simulink model "Model_plant"  (R2022a)
settings: Solver=VariableStepAuto  StartTime=0.0  StopTime=10  RelTol=1e-3
values from neighbouring files (symbols this model uses):
  init = [theta_m_init; theta_l_init; thetadot_m_init; thetadot_l_init; Ia_init]    [ELEN90064_Project_Parameters.m]
undefined symbols (not defined in the file or in its folder): denC, denG, numC, numG
settings Model: Creator=Admin  LastModifiedBy=yang

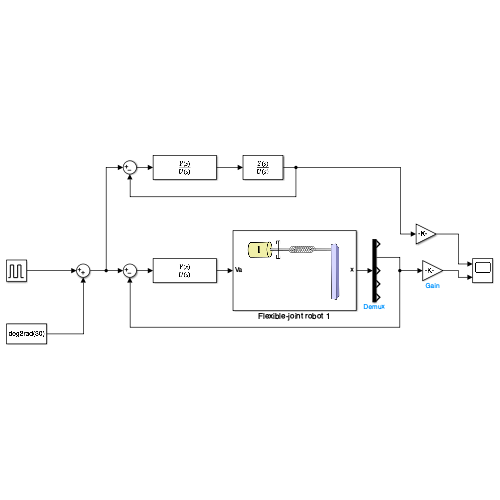
[thumbnail: Simulink's stored preview of the top-level diagram]
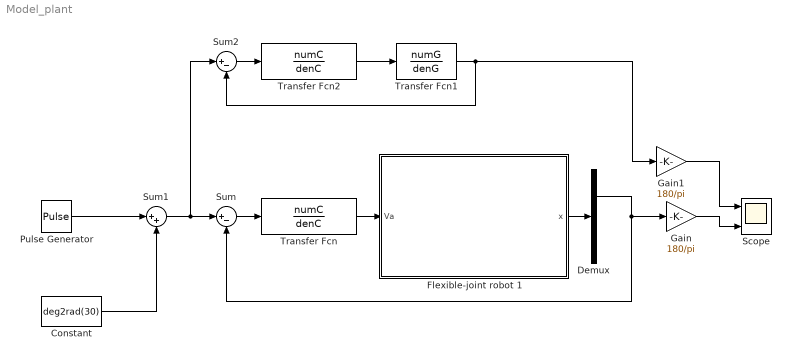
== system Model_plant ==
  Constant : Constant  Value=deg2rad(30)
  Demux : Demux  Outputs=5
  Flexible-joint robot 1 : Subsystem
      mask Display: image('$imagefile'); % Use "Edit Image" on toolstrip to change.
  Gain : Gain  Gain=180/pi
  Gain1 : Gain  Gain=180/pi
  Pulse Generator : DiscretePulseGenerator  PulseType=Time based  Amplitude=deg2rad(30)  Period=5  PulseWidth=50
  Scope : Scope  NumInputPorts=2
  Sum : Sum  Inputs=|+-
  Sum1 : Sum  Inputs=|++
  Sum2 : Sum  Inputs=|+-
  Transfer Fcn : TransferFcn  Numerator=numC  Denominator=denC
  Transfer Fcn1 : TransferFcn  Numerator=numG  Denominator=denG
  Transfer Fcn2 : TransferFcn  Numerator=numC  Denominator=denC
  wires:
  Sum/1 -> Transfer Fcn/1
  Pulse Generator/1 -> Sum1/1
  Constant/1 -> Sum1/2
  Gain/1 -> Scope/2
  Transfer Fcn/1 -> Flexible-joint robot 1/1(Va)
  Flexible-joint robot 1/1(x) -> Demux/1
  Demux/2 -> Gain/1, Sum/2
  Transfer Fcn1/1 -> Gain1/1, Sum2/2
  Sum1/1 -> Sum2/1, Sum/1
  Sum2/1 -> Transfer Fcn2/1
  Transfer Fcn2/1 -> Transfer Fcn1/1
  Gain1/1 -> Scope/1

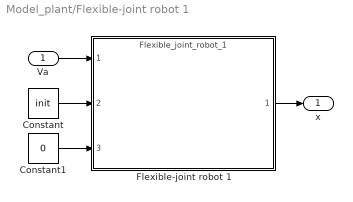
== system Model_plant/Flexible-joint robot 1 ==
  Va : Inport
  Constant : Constant  Value=init
  Constant1 : Constant  Value=0
  Flexible-joint robot 1 : ModelReference  ModelNameDialog=Flexible_joint_robot_1  ModelReferenceVersion=1.63  CopyOfModelProtected=on
  x : Outport
  wires:
  Constant/1 -> Flexible-joint robot 1/2
  Constant1/1 -> Flexible-joint robot 1/3
  Flexible-joint robot 1/1 -> x/1
  Va/1 -> Flexible-joint robot 1/1
